simulink model "UAV_Research_Environment"  (R2025a)
settings: Solver=ode23t  StartTime=0.0  StopTime=130  MaxStep=2e-3  RelTol=1e-4  AbsTol=1e-3  EnableMultiTasking=on
InitFcn:
  | skipInitialization = false;
  | 
  | if evalin('base', ...
  |         'exist(''CONTROLLER_TUNING_ACTIVE'',''var'')')
  | 
  |     skipInitialization = evalin('base', ...
  |         'logical(CONTROLLER_TUNING_ACTIVE)');
  | end
  | 
  | if ~skipInitialization
  | 
  |     icraControllerPrepared = false;
  | 
  |     hasICRAVariables = evalin('base', ...
  |         ['exist(''AUTOPILOT'',''var'') && ' ...
  |          'exist(''ICRA_ACTIVE_CONTROLLER'',''var'') && ' ...
  |          'exist(''ICRA_ACTIVE_RUN_ID'',''var'')']);
  | 
  |     if hasICRAVariables
  | 
  |         icraControllerPrepared = evalin('base', ...
  |             ['isstruct(AUTOPILOT) && ' ...
  |              'isfield(AUTOPILOT,''info'') && ' ...
  |              'isfield(AUTOPILOT.info,''ICRAControllerID'') && ' ...
  |              'strcmp(string(AUTOPILOT.info.ICRAControllerID), ' ...
  |                     'string(ICRA_ACTIVE_CONTROLLER))']);
  | 
  |     end
  | 
  |     if icraControllerPrepared
  |         skipInitialization = true;
  |     end
  | end
  | 
  | if ~skipInitialization
  | 
  |     mdl = bdroot;
  | 
  |     mdl_file = get_param(mdl, 'FileName');
  | 
  |     project_root = fileparts(mdl_file);
  | 
  |     init_file = fullfile(project_root, 'initialize_project.m');
  | 
  |     if exist(init_file, 'file')
  | 
  |         run(init_file);
  | 
  |     else
  | 
  |         error('initialize_project.m was not found in the model folder.');
  | 
  |     end
  | end
values from neighbouring files (symbols this model uses):
  A_UAV = struct()    [UAV_analytical.m]
  AUTOPILOT = struct()    [UAV_autopilot.m]
  B_UAV = struct()    [UAV_block.m]
  D = A_UAV.source.propeller_diameter_m    [UAV_analytical.m]    (also in plot_controller_results.m = permute(                  D,                  order); plot_estimator_results.m = permute(              D,              order); plot_mission_results.m = permute(                  D,                  order); plot_touchdown_diagnostics.m = permute(                  D,                  order))
  OPERATOR_MODE = OPERATOR_MODE_MANUAL    [initialize_project.m]    (also in uav_remote_gui.m = uint8(0))
  P_ENV = struct()    [Environment.m]
  P_UAV = struct()    [UAV_simscape.m]
  s = sin(angle)    [uav_remote_gui.m]
  SENSOR = struct()    [UAV_sensors.m]
  TRAJECTORY_CONFIG = struct()    [UAV_trajectories.m]
  TRAJECTORY_ID = uint8(          trajectoryIDNumeric)    [UAV_trajectories.m]
  X = reshape(                  D,                  nt,                  [])    [plot_controller_results.m]    (also in plot_estimator_results.m = reshape(              D,              nt,              []); plot_mission_results.m; plot_touchdown_diagnostics.m; plot_trajectory_3d.m)
  Y = absolutePlanNED(1,:)    [plot_trajectory_3d.m]    (also in uav_remote_gui.m = positionNED(:,1))
  Z = landedCGDown -          absolutePlanNED(3,:)    [plot_trajectory_3d.m]    (also in uav_remote_gui.m = landedCGDown-positionNED(:,3))
undefined symbols (not defined in the file or in its folder): Acceleration_ref, F, fractalcoef, Light, MIL, Position_ref, Velocity_ref, Yaw_ref, YawRate_ref
libraries: sm_lib x49, nesl_utility x29, fl_lib x17, slpidlib x16, simulink x14, ee_lib x5, sdl_lib x4, aerolibwind2 x3, aerolibatmos2 x2, sensorbarometerlib x1, sensorgpslib x1, mspsensorlib x1
(part 1 of 9)
settings Model: ModifiedByFormat=Anonymous  Creator=Anonymous  LastModifiedBy=Anonymous
settings SolverCC: AutoScaleAbsTol=off  ZeroCrossAlgorithm=Adaptive  MaxZcPerStep=1.0
settings DataIOCC: LimitDataPoints=on  MaxDataPoints=10000  DSMLogging=off
settings OptimizationCC: ReuseModelBlockBuffer=off  LifeSpan=inf
settings DebuggingCC: AlgebraicLoopMsg=none  IgnoredZcDiagnostic=none  UnconnectedInputMsg=warning  UnconnectedOutputMsg=warning  UnconnectedLineMsg=warning  AllowSymbolicDim=off  SubsystemReferenceDiagnosticForUnitTest=warning  SFUnexpectedBacktrackingDiag=warning  SFNoUnconditionalDefaultTransitionDiag=warning  SFExecutionAtInitializationDiag=none  ArithmeticOperatorsInVariantConditions=warning
settings ModelReferenceCC: EnableRefExpFcnMdlSchedulingChecks=on
settings SFSimCC: SimUseLocalCustomCode=off  CustomCodeUndefinedFunction=UseInterfaceOnly
settings RTWCC: RTWUseLocalCustomCode=off  GPUComputeCapability=3.5  DLArmComputeVersion=19.05
settings CodeAppCC: StateflowObjectComments=on
settings GRTTargetCC: TargetLangStandard=C89/C90 (ANSI)
settings ConfigComp: CovMetricSettings=dw  CovSaveCumulativeToWorkspaceVar=on  CovSaveSingleToWorkspaceVar=on  CovExternalEMLEnable=off  CovSFcnEnable=off
settings SimscapeCC: SimscapeLogDataHistory=10000.0
settings ExplorerConfigSet: InternalSimMechanicsExplorerSettings=|
  | <ExplorerConfiguration>
  | 
  |   <canonicalview>default</canonicalview>
  | 
  |   <TilePanel>
  |     <TileInfo>
  |       <Tiles Columns="1" Count="1" Height="815" Rows="1" Width="1140">
  |         <Row Weight="1"/>
  |         <Column Weight="1"/>
  |         <Tile Height="1" Width="1" X="0" Y="0"/>
  |       </Tiles>
  |     </TileInfo>
  |     <SceneInfo>
  |       <SceneViewer>
  |         <IsThisViewStd>
  |           <IsStandardView>off</IsStandardView>
  |           <StandardViewName>Front</StandardViewName>
  |         </IsThisViewStd>
  |         <BGColor>
  |           <R>1</R>
  |           <G>1</G>
  |           <B>1</B>
  |           <A>1</A>
  |         </BGColor>
  |         <Camera>
  |           <DoPerspective>off</DoPerspective>
  |           <Position>
  |             <X>0.72021697851709687</X>
  |             <Y>23.914268823911655</Y>
  |             <Z>0.9247861603673575</Z>
  |           </Position>
  |           <Center>
  |             <X>0.72021697851709687</X>
  |             <Y>0.79760772389431911</Y>
  |             <Z>0.9247861603673575</Z>
  |           </Center>
  |           <Up>
  |             <X>0</X>
  |             <Y>0</Y>
  |             <Z>1</Z>
  |           </Up>
  |           <XLim>3.1326972550118835</XLim>
  |           <YLim>3.1326972550118835</YLim>
  |           <ViewLimDist>0.01</ViewLimDist>
  |         </Camera>
  |       </SceneViewer>
  |     </SceneInfo>
  |   </TilePanel>
  | 
  |   <MechEditorPanel>
  |     <GfxPanelCameraMap/>
  |     <Cameras/>
  |     <VideoCreator>
  |       <IncludeTiles>All</IncludeTiles>
  |       <IncludeTime>on</IncludeTime>
  |       <IncludeWorldFrame>off</IncludeWorldFrame>
  |       <PlaybackSpeedRatio>1</PlaybackSpeedRatio>
  |       <FrameRate>30</FrameRate>
  |       <FrameSize>auto</FrameSize>
  |       <VideoFormat>UncompressedAVI</VideoFormat>
  |     </VideoCreator>
  |   </MechEditorPanel>
  | 
  |   <PlaybackSettings>
  |     <PlaybackSpeedFactor>1</PlaybackSpeedFactor>
  |   </PlaybackSettings>
  | 
  | </ExplorerConfiguration>

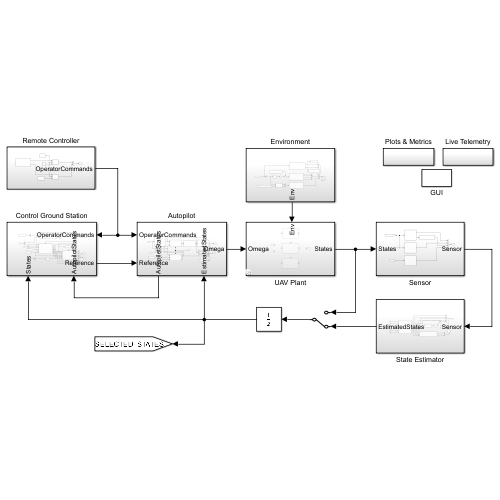
[thumbnail: Simulink's stored preview of the top-level diagram]
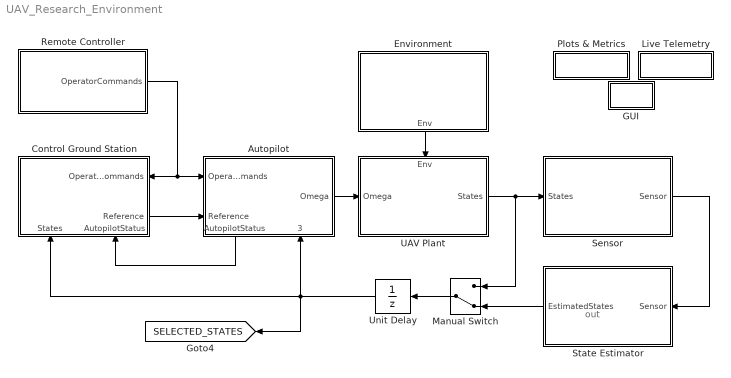
== system UAV_Research_Environment ==
  note: out
  Autopilot : Subsystem
      settings: PortSchema="{\"entries\":[{\"content\":{\"sides\":[{\"content\":{\"connectorIds\":[\"In1\",\"In2\"]},\"type\":\"ConnectorPlacement.EquallySpacedRectSide\",\"uuid\":\"e70f1091-d358-4451-85c8-8eba7ccb6162\"},{\"content\":{\"connectorIds\":[\"Out1\"],\"side\":\"RIGHT\"},\"type\":\"ConnectorPlacement.EquallySpacedRectSide\",\"uuid\":\"2dd7087d-b972-437c-8483-21f370874524\"},{\"content\":{\"side\":\"TOP\"},\"type\":\"ConnectorPlacement.EquallySpacedRectSide\",\"uuid\":\"61fa1c6d-d900-4918-8b03-2266ce99a694\"},{\"content\":{\"connectorIds\":[\"Out2\",\"In3\"],\"side\":\"BOTTOM\"},\"type\":\"ConnectorPlacement.EquallySpacedRectSide\",\"uuid\":\"0a489e47-d763-416d-8560-669941892c49\"}]},\"type\":\"ConnectorPlacement.EquallySpacedConnector\",\"uuid\":\"bc420e13-87ad-4ba2-aca7-0668641bff4a\"}],\"packageUris\":[\"http://schema.mathworks.com/mf0/Connector/R2020b\"],\"version\":\"1.0\"}"
  Control Ground Station : Subsystem
      settings: PortSchema="{\"entries\":[{\"content\":{\"sides\":[{\"content\":{},\"type\":\"ConnectorPlacement.EquallySpacedRectSide\",\"uuid\":\"136384be-95d6-4553-ba03-2aeaf9dd8964\"},{\"content\":{\"connectorIds\":[\"In3\",\"Out1\"],\"side\":\"RIGHT\"},\"type\":\"ConnectorPlacement.EquallySpacedRectSide\",\"uuid\":\"258859f6-93b5-427a-ab6d-3a33e6d3f50d\"},{\"content\":{\"side\":\"TOP\"},\"type\":\"ConnectorPlacement.EquallySpacedRectSide\",\"uuid\":\"470d9523-0035-468d-b4f0-7ce4b4aa87dd\"},{\"content\":{\"connectorIds\":[\"In1\",\"In2\"],\"side\":\"BOTTOM\"},\"type\":\"ConnectorPlacement.EquallySpacedRectSide\",\"uuid\":\"eb9250ba-ba34-48b7-bfa4-7567789009ef\"}]},\"type\":\"ConnectorPlacement.EquallySpacedConnector\",\"uuid\":\"8818c9e9-852d-490b-83ee-80294e50417b\"}],\"packageUris\":[\"http://schema.mathworks.com/mf0/Connector/R2020b\"],\"version\":\"1.0\"}"
  Environment : Subsystem
      settings: PortSchema="{\"entries\":[{\"content\":{\"sides\":[{\"content\":{},\"type\":\"ConnectorPlacement.EquallySpacedRectSide\",\"uuid\":\"20d534b3-ad30-4c14-921c-ffe2bc2505b4\"},{\"content\":{\"side\":\"RIGHT\"},\"type\":\"ConnectorPlacement.EquallySpacedRectSide\",\"uuid\":\"42e7d556-7bdf-4888-9f8c-71685b18f3c6\"},{\"content\":{\"side\":\"TOP\"},\"type\":\"ConnectorPlacement.EquallySpacedRectSide\",\"uuid\":\"98b28398-80a3-4874-ba79-5e078ee713b6\"},{\"content\":{\"connectorIds\":[\"Out1\"],\"side\":\"BOTTOM\"},\"type\":\"ConnectorPlacement.EquallySpacedRectSide\",\"uuid\":\"66822910-7c6b-4720-98d4-5d952560352f\"}]},\"type\":\"ConnectorPlacement.EquallySpacedConnector\",\"uuid\":\"f342a492-18c2-4fcb-af45-73348ac80d72\"}],\"packageUris\":[\"http://schema.mathworks.com/mf0/Connector/R2020b\"],\"version\":\"1.0\"}"
  GUI : Subsystem
      settings: OpenFcn=|
      | mdl = bdroot(gcb);
      | mdlFolder = fileparts(get_param(mdl,'FileName'));
      | 
      | oldFolder = pwd;
      | cleanupObj = onCleanup(@() cd(oldFolder));
      | 
      | cd(mdlFolder);
      | uav_remote_gui(mdl);
  Live Telemetry : Subsystem
  Manual Switch : ManualSwitch  CurrentSetting=0
  Plots & Metrics : Subsystem
  Remote Controller : Subsystem
  Sensor : Subsystem
  State Estimator : Subsystem
      settings: PortSchema="{\"entries\":[{\"content\":{\"sides\":[{\"content\":{\"connectorIds\":[\"Out1\"]},\"type\":\"ConnectorPlacement.EquallySpacedRectSide\",\"uuid\":\"59a621b8-c7fd-4210-ae06-7e4287b99fe9\"},{\"content\":{\"connectorIds\":[\"In1\"],\"side\":\"RIGHT\"},\"type\":\"ConnectorPlacement.EquallySpacedRectSide\",\"uuid\":\"3b6e64c1-8f25-466d-be87-51a5dfb932f3\"},{\"content\":{\"side\":\"TOP\"},\"type\":\"ConnectorPlacement.EquallySpacedRectSide\",\"uuid\":\"7168969e-7eff-41f7-8f21-8d68bf623552\"}]},\"type\":\"ConnectorPlacement.EquallySpacedConnector\",\"uuid\":\"8e25eed9-214a-4c11-975e-8e28997d468c\"}],\"packageUris\":[\"http://schema.mathworks.com/mf0/Connector/R2020b\"],\"version\":\"1.0\"}"
  UAV Plant : Subsystem  Variant=on  AllowFlexibleInterface=off
      settings: PortSchema="{\"entries\":[{\"content\":{\"sides\":[{\"content\":{\"connectorIds\":[\"In1\"]},\"type\":\"ConnectorPlacement.EquallySpacedRectSide\",\"uuid\":\"3610bc50-1c95-4e4a-95b0-008058f44424\"},{\"content\":{\"connectorIds\":[\"Out1\"],\"side\":\"RIGHT\"},\"type\":\"ConnectorPlacement.EquallySpacedRectSide\",\"uuid\":\"eac11400-6209-4713-b6ed-f17afc459a7e\"},{\"content\":{\"connectorIds\":[\"In2\"],\"side\":\"TOP\"},\"type\":\"ConnectorPlacement.EquallySpacedRectSide\",\"uuid\":\"1cd5a0d1-33ba-4090-85ff-88440ab8bf38\"}]},\"type\":\"ConnectorPlacement.EquallySpacedConnector\",\"uuid\":\"d77e6d8a-bf97-49e4-8cac-05db6bcacb57\"}],\"packageUris\":[\"http://schema.mathworks.com/mf0/Connector/R2020b\"],\"version\":\"1.0\"}"
  Unit Delay : UnitDelay  SampleTime=-1  HasFrameUpgradeWarning=on
  tag scope: SELECTED_STATES=global
  wires:
  UAV Plant/1(States) -> Sensor/1(States), Manual Switch/1
  Sensor/1(Sensor) -> State Estimator/1(Sensor)
  Control Ground Station/1(Reference) -> Autopilot/2(Reference)
  Remote Controller/1(OperatorCommands) -> Control Ground Station/3(OperatorCommands), Autopilot/1(OperatorCommands)
  Autopilot/2(AutopilotStatus) -> Control Ground Station/2(AutopilotStatus)
  Manual Switch/1 -> Unit Delay/1
  Unit Delay/1 -> Control Ground Station/1(States), Autopilot/3(EstimatedStates), [SELECTED_STATES]
  State Estimator/1(EstimatedStates) -> Manual Switch/2
  Autopilot/1(Omega) -> UAV Plant/1(Omega)
  Environment/1(Env) -> UAV Plant/2(Env)

== system UAV_Research_Environment/Autopilot ==
  OperatorCommands : Inport
  Reference : Inport  Port=2
  EstimatedStates : Inport  Port=3
  Bus Creator : BusCreator  Inputs=5
  Bus Selector : BusSelector  OutputSignals=mode,armed,reset,missionComplete
  Control Allocation : Subsystem
  Flight Control : Subsystem
      settings: PortSchema="{\"entries\":[{\"content\":{\"sides\":[{\"content\":{\"connectorIds\":[\"In1\",\"In2\"]},\"type\":\"ConnectorPlacement.EquallySpacedRectSide\",\"uuid\":\"f0a7248d-f68a-4ef2-8432-35dfc7f6e14f\"},{\"content\":{\"connectorIds\":[\"Out1\"],\"side\":\"RIGHT\"},\"type\":\"ConnectorPlacement.EquallySpacedRectSide\",\"uuid\":\"efba777c-49ac-415f-93a0-e17947ba5c8f\"},{\"content\":{\"side\":\"TOP\"},\"type\":\"ConnectorPlacement.EquallySpacedRectSide\",\"uuid\":\"6197b28d-1ee2-4df8-818f-0bd555e896ae\"},{\"content\":{\"connectorIds\":[\"In3\"],\"side\":\"BOTTOM\"},\"type\":\"ConnectorPlacement.EquallySpacedRectSide\",\"uuid\":\"82eb3d58-e8e8-4a8e-8208-c30c9bf3b54b\"}]},\"type\":\"ConnectorPlacement.EquallySpacedConnector\",\"uuid\":\"801f385a-c387-4f85-8315-b8cc9b2ee46f\"}],\"packageUris\":[\"http://schema.mathworks.com/mf0/Connector/R2020b\"],\"version\":\"1.0\"}"
  Flight Management : Subsystem
      settings: PortSchema="{\"entries\":[{\"content\":{\"sides\":[{\"content\":{\"connectorIds\":[\"In1\"]},\"type\":\"ConnectorPlacement.EquallySpacedRectSide\",\"uuid\":\"cd28ed6d-ec01-4006-9fc1-ea9cf3b5ab9c\"},{\"content\":{\"connectorIds\":[\"Out1\"],\"side\":\"RIGHT\"},\"type\":\"ConnectorPlacement.EquallySpacedRectSide\",\"uuid\":\"9cadd399-a218-43e8-9df1-ffad97f9a650\"},{\"content\":{\"side\":\"TOP\"},\"type\":\"ConnectorPlacement.EquallySpacedRectSide\",\"uuid\":\"feac389c-df1b-4914-811b-4035f0dee4d7\"},{\"content\":{\"connectorIds\":[\"In2\",\"In3\",\"In4\",\"In5\"],\"side\":\"BOTTOM\"},\"type\":\"ConnectorPlacement.EquallySpacedRectSide\",\"uuid\":\"4a7ea741-3b46-4c9a-969c-f6d865221263\"}]},\"type\":\"ConnectorPlacement.EquallySpacedConnector\",\"uuid\":\"336e0f35-9a21-4036-b176-5dadcac79355\"}],\"packageUris\":[\"http://schema.mathworks.com/mf0/Connector/R2020b\"],\"version\":\"1.0\"}"
  Landed Detector : Subsystem
      settings: PortSchema="{\"entries\":[{\"content\":{\"sides\":[{\"content\":{\"connectorIds\":[\"In1\",\"In2\",\"In3\"]},\"type\":\"ConnectorPlacement.EquallySpacedRectSide\",\"uuid\":\"9d9528e8-7e55-467e-913b-dcdc8299219a\"},{\"content\":{\"connectorIds\":[\"Out1\",\"Out2\"],\"side\":\"RIGHT\"},\"type\":\"ConnectorPlacement.EquallySpacedRectSide\",\"uuid\":\"a2ddb638-2a20-4bf0-9798-8e8fe050fb6e\"},{\"content\":{\"connectorIds\":[\"In4\"],\"side\":\"TOP\"},\"type\":\"ConnectorPlacement.EquallySpacedRectSide\",\"uuid\":\"4b4cf5b5-d356-42f7-9123-fe3c672c98b7\"}]},\"type\":\"ConnectorPlacement.EquallySpacedConnector\",\"uuid\":\"5fd14821-3580-4c60-a331-c7350594f720\"}],\"packageUris\":[\"http://schema.mathworks.com/mf0/Connector/R2020b\"],\"version\":\"1.0\"}"
  Motor Command : Subsystem
      settings: PortSchema="{\"entries\":[{\"content\":{\"sides\":[{\"content\":{\"connectorIds\":[\"In1\"]},\"type\":\"ConnectorPlacement.EquallySpacedRectSide\",\"uuid\":\"f0a7248d-f68a-4ef2-8432-35dfc7f6e14f\"},{\"content\":{\"connectorIds\":[\"Out1\"],\"side\":\"RIGHT\"},\"type\":\"ConnectorPlacement.EquallySpacedRectSide\",\"uuid\":\"efba777c-49ac-415f-93a0-e17947ba5c8f\"},{\"content\":{\"connectorIds\":[\"In2\"],\"side\":\"TOP\"},\"type\":\"ConnectorPlacement.EquallySpacedRectSide\",\"uuid\":\"6197b28d-1ee2-4df8-818f-0bd555e896ae\"}]},\"type\":\"ConnectorPlacement.EquallySpacedConnector\",\"uuid\":\"801f385a-c387-4f85-8315-b8cc9b2ee46f\"}],\"packageUris\":[\"http://schema.mathworks.com/mf0/Connector/R2020b\"],\"version\":\"1.0\"}"
  Omega : Outport
  AutopilotStatus : Outport  Port=2
  tag scope: AUTOPILOT_ST=global, OMEGA=global
  wires:
  Flight Control/1(FlightControl) -> Control Allocation/1(FlightControl)
  Control Allocation/1(MotorCmd) -> Motor Command/1(MotorCmd)
  Motor Command/1(Omega) -> Omega/1, [OMEGA]
  Flight Management/1(FlightManagement) -> Bus Selector/1, Motor Command/2(FlightManagement), Flight Control/1(FlightManagement)
  Reference/1 -> Landed Detector/1(Reference), Flight Control/2(Reference), Flight Management/1(Reference)
  EstimatedStates/1 -> Flight Control/3(EstimatedStates), Landed Detector/4(EstimatedStates)
  OperatorCommands/1 -> Landed Detector/3(OperatorCommands), Flight Management/3(OperatorCommands)
  Landed Detector/1(Landed) -> Flight Management/2(Landed), Bus Creator/5  "Landed"
  Bus Selector/1 -> Bus Creator/1  "<mode>"
  Bus Selector/2 -> Bus Creator/2  "<armed>"
  Bus Selector/3 -> Bus Creator/3  "<reset>"
  Bus Selector/4 -> Bus Creator/4  "<missionComplete>"
  Bus Creator/1 -> [AUTOPILOT_ST], AutopilotStatus/1
  [EST_STATUS] -> Flight Management/4(EstimatorStatus), Landed Detector/2(EstimatorStatus)
  Landed Detector/2(TouchdownCandidate) -> Flight Management/5(TouchdownCandidate)

== system UAV_Research_Environment/Control Ground Station ==
  States : Inport
  AutopilotStatus : Inport  Port=2
  OperatorCommands : Inport  Port=3
  Bus Creator : BusCreator  Inputs=8
  Bus Selector : BusSelector  OutputSignals=ArmCommand,RunTrajectoryRequestID
  Bus Selector1 : BusSelector  OutputSignals=Position,Velocity
  Bus Selector2 : BusSelector  OutputSignals=Landed
  Bus Selector3 : BusSelector  OutputSignals=Position
  "Digital Clock " : DigitalClock  SampleTime=AUTOPILOT.rate.controlSampleTime_s
  Home Manager : MATLAB Function  TreatAsAtomicUnit=on
  Mission Manager : Subsystem
      settings: PortSchema="{\"entries\":[{\"content\":{\"sides\":[{\"content\":{\"connectorIds\":[\"In1\",\"In2\",\"In3\",\"In4\",\"In5\",\"In6\"]},\"type\":\"ConnectorPlacement.EquallySpacedRectSide\",\"uuid\":\"bc5e4697-56b9-4dea-9e35-80b1d53c2be1\"},{\"content\":{\"connectorIds\":[\"Out1\",\"Out2\",\"Out3\",\"Out4\",\"Out5\",\"Out6\"],\"side\":\"RIGHT\"},\"type\":\"ConnectorPlacement.EquallySpacedRectSide\",\"uuid\":\"fb3706cb-7914-4411-8945-e3646c2cb779\"},{\"content\":{\"connectorIds\":[\"In7\"],\"side\":\"TOP\"},\"type\":\"ConnectorPlacement.EquallySpacedRectSide\",\"uuid\":\"dbed3f0a-ac38-4c4a-aeac-a7a9b73a6d14\"}]},\"type\":\"ConnectorPlacement.EquallySpacedConnector\",\"uuid\":\"9e38a936-7e60-4815-89b3-1f8eea1eae0e\"}],\"packageUris\":[\"http://schema.mathworks.com/mf0/Connector/R2020b\"],\"version\":\"1.0\"}"
  Mission Plan : Subsystem
  Terminator : Terminator
  Unit Delay : UnitDelay  InitialCondition=false  SampleTime=0.005  HasFrameUpgradeWarning=on
  Waypoint Navigator : Subsystem
      settings: PortSchema="{\"entries\":[{\"content\":{\"sides\":[{\"content\":{\"connectorIds\":[\"In1\",\"In2\",\"In3\",\"In4\",\"In5\",\"In6\",\"In7\"]},\"type\":\"ConnectorPlacement.EquallySpacedRectSide\",\"uuid\":\"a5c6b6ee-d5d5-4725-a074-dc49922cc7be\"},{\"content\":{\"connectorIds\":[\"Out1\",\"Out2\",\"Out3\",\"Out4\",\"Out5\"],\"side\":\"RIGHT\"},\"type\":\"ConnectorPlacement.EquallySpacedRectSide\",\"uuid\":\"658ed11c-ff5e-46da-8e6b-259d14db485f\"},{\"content\":{\"connectorIds\":[\"In8\"],\"side\":\"TOP\"},\"type\":\"ConnectorPlacement.EquallySpacedRectSide\",\"uuid\":\"7f46b370-90bd-452a-8751-2617752800df\"}]},\"type\":\"ConnectorPlacement.EquallySpacedConnector\",\"uuid\":\"a0f43945-89fe-4e34-a980-6cf45089d260\"}],\"packageUris\":[\"http://schema.mathworks.com/mf0/Connector/R2020b\"],\"version\":\"1.0\"}"
  Reference : Outport
  tag scope: CGS=global, MISSION_PLAN=global, NUM_WAYPOINTS=global
  wires:
  OperatorCommands/1 -> Bus Selector/1
  Bus Selector/2 -> Mission Manager/1(RunTrajectoryRequestID)  "<RunTrajectoryRequestID>"
  States/1 -> Bus Selector1/1
  Bus Selector1/2 -> Mission Manager/3(Velocity)  "<Velocity>"
  "Digital Clock "/1 -> Waypoint Navigator/1(t), Mission Manager/6(t)
  Bus Selector1/1 -> Mission Manager/2(Position)  "<Position>"
  Mission Manager/1(TargetPosition) -> Waypoint Navigator/3(TargetPosition)
  Mission Manager/2(TargetYaw) -> Waypoint Navigator/4(TargetYaw)
  Mission Manager/3(TargetID) -> Waypoint Navigator/5(TargetID)
  Bus Creator/1 -> [CGS], Reference/1
  Waypoint Navigator/1(Position_ref) -> Bus Creator/1
  Waypoint Navigator/2(Velocity_ref) -> Bus Creator/2
  Waypoint Navigator/3(Acceleration_ref) -> Bus Creator/3
  Waypoint Navigator/4(Yaw_ref) -> Bus Creator/4
  Waypoint Navigator/5(YawRate_ref) -> Bus Creator/5
  Mission Manager/4(Phase) -> Bus Creator/6, Waypoint Navigator/6(Phase)
  Mission Manager/5(Active) -> Bus Creator/7
  Mission Manager/6(Complete) -> Bus Creator/8
  AutopilotStatus/1 -> Bus Selector2/1
  Bus Selector2/1 -> Unit Delay/1  "<Landed>"
  Unit Delay/1 -> Waypoint Navigator/7(Landed)
  Bus Selector/1 -> Home Manager/2(ArmCommand)  "<ArmCommand>"
  Home Manager/1(HomePosition) -> Mission Plan/1(HomePosition)
  [EST_STATUS] -> Mission Manager/4(EstimatorStatus)
  Mission Plan/1(MissionPlan) -> Waypoint Navigator/2(MissionPlan), [MISSION_PLAN], Mission Manager/7(MissionPlan)
  [TRUE_STATES] -> Bus Selector3/1
  Bus Selector3/1 -> Home Manager/1(HomePositionSource)  "<Position>"
  Mission Plan/2(NumWaypoints) -> [NUM_WAYPOINTS], Waypoint Navigator/8(NumWaypoints), Mission Manager/5(NumWaypoints)
  Home Manager/2(HomeValid) -> Terminator/1

== system UAV_Research_Environment/Environment ==
  Atmosphere : aerolibatmos2/ISA Atmosphere Model  useExtended=off  action=None  custom=off  viscosityOut=off  g=9.80665  gamma=1.4  R=287.0531  L=0.0065  h_trop=11000  h_strat=20000  rho0=1.225  P0=101325  T0=288.15  h0=0  S=110.4  Tref=273.15  muref=1.716e-5
  Bus Creator : BusCreator  Inputs=3
  Bus Creator1 : BusCreator  Inputs=2
  Bus Creator2 : BusCreator  Inputs=4
  Bus Selector2 : BusSelector  OutputSignals=Position
  Constant : Constant  Value=P_ENV.location.altitude_ref_m
  Constant1 : Constant  Value=P_ENV.location.flat_earth_href_m
  Flat Earth to LLA : FlatEarth2LLA  LL0=[P_ENV.location.latitude_ref_deg P_ENV.location.longitude_ref_deg]  psi=P_ENV.location.heading_ref_deg
  Gain : Gain  Gain=-1
  Gravity : GravityWGS84
  Selector : Selector  InputPortWidth=3  IndexOptions=Index vector (dialog)  Indices=3  OutputSizes=1
  Sum : Sum  Inputs=++|
  To Workspace : ToWorkspace  VariableName=windVelocityLog  SaveFormat=Timeseries  SampleTime=-1
  To Workspace1 : ToWorkspace  VariableName=windAngularVelocityLog  SaveFormat=Timeseries  SampleTime=-1
  Vector Concatenate1 : Concatenate
  Wind Disturbances : Subsystem  Variant=on
  Env : Outport
  tag scope: ENV=global
  wires:
  Gain/1 -> Sum/2
  Wind Disturbances/1(v_wind) -> Bus Creator1/1, To Workspace/1  "v"
  Atmosphere/1 -> Bus Creator2/1  "Temperature"
  Atmosphere/2 -> Bus Creator2/2  "SoundSpeed"
  Atmosphere/4 -> Bus Creator2/4  "AirDensity"
  Atmosphere/3 -> Bus Creator2/3  "AirPressure"
  Gravity/1 -> Bus Creator/3  "Gravity"
  [TRUE_STATES] -> Wind Disturbances/1(States), Bus Selector2/1
  Constant1/1 -> Flat Earth to LLA/2
  Flat Earth to LLA/1 -> Vector Concatenate1/1
  Flat Earth to LLA/2 -> Vector Concatenate1/2
  Vector Concatenate1/1 -> Gravity/1
  Bus Selector2/1 -> Selector/1, Flat Earth to LLA/1  "<Position>"
  Wind Disturbances/2(w_wind) -> Bus Creator1/2, To Workspace1/1  "w"
  Selector/1 -> Gain/1  "z"
  Bus Creator/1 -> Env/1, [ENV]
  Bus Creator2/1 -> Bus Creator/2  "Atmosphere"
  Bus Creator1/1 -> Bus Creator/1  "Wind"
  Sum/1 -> Atmosphere/1
  Constant/1 -> Sum/1

== system UAV_Research_Environment/GUI ==

== system UAV_Research_Environment/Live Telemetry ==
  Bus Selector : BusSelector  OutputSignals=Phase,Active,Complete,Position_ref
  Bus Selector1 : BusSelector  OutputSignals=Position,Attitude.Euler
  Bus Selector2 : BusSelector  OutputSignals=mode,armed,missionComplete,Landed
  Bus Selector3 : BusSelector  OutputSignals=Position,Attitude.Euler
  Bus Selector4 : BusSelector  OutputSignals=Position
  "Digital Clock " : DigitalClock  SampleTime=AUTOPILOT.rate.controlSampleTime_s
  Telemetry_Pack : MATLAB Function  TreatAsAtomicUnit=on
  To Workspace : ToWorkspace  VariableName=liveTelemetryLog  SaveFormat=Timeseries  SampleTime=-1
  wires:
  [CGS] -> Bus Selector/1
  [SELECTED_STATES] -> Bus Selector1/1
  [AUTOPILOT_ST] -> Bus Selector2/1
  "Digital Clock "/1 -> Telemetry_Pack/1(t)
  Bus Selector/1 -> Telemetry_Pack/2(Phase)  "<Phase>"
  Bus Selector/2 -> Telemetry_Pack/3(Active)  "<Active>"
  Bus Selector/3 -> Telemetry_Pack/4(Complete)  "<Complete>"
  Bus Selector/4 -> Telemetry_Pack/5(Position_ref)  "<Position_ref>"
  Bus Selector1/1 -> Telemetry_Pack/10(Position)  "<Position>"
  Bus Selector2/1 -> Telemetry_Pack/6(mode)  "<mode>"
  Bus Selector2/2 -> Telemetry_Pack/7(armed)  "<armed>"
  Bus Selector2/3 -> Telemetry_Pack/8(missionComplete)  "<missionComplete>"
  Bus Selector2/4 -> Telemetry_Pack/9(Landed)  "<Landed>"
  Telemetry_Pack/1(Telemetry) -> To Workspace/1
  [MISSION_PLAN] -> Telemetry_Pack/13(MissionPlan)
  [OMEGA] -> Telemetry_Pack/12(MotorSpeeds)
  Bus Selector1/2 -> Telemetry_Pack/11(Euler)  "<Euler>"
  [TRUE_STATES] -> Bus Selector3/1
  [EST_STATES] -> Bus Selector4/1
  Bus Selector4/1 -> Telemetry_Pack/16(EstPosition)  "<Position>"
  Bus Selector3/2 -> Telemetry_Pack/15(TrueEuler)  "<Euler>"
  Bus Selector3/1 -> Telemetry_Pack/14(TruePosition)  "<Position>"
  [NUM_WAYPOINTS] -> Telemetry_Pack/17(NumWaypoints)

== system UAV_Research_Environment/Plots & Metrics ==
  Data Logging : Subsystem
  Estimator Comparison : Subsystem
  wires:
  [TRUE_STATES] -> Data Logging/3(TrueStates), Estimator Comparison/1(True)
  [EST_STATES] -> Data Logging/2(EstStates), Estimator Comparison/2(Est)
  Estimator Comparison/1(EstimatorComparison) -> Data Logging/1(EstimatorComparison)
  [CGS] -> Data Logging/7(CGS)
  [OMEGA] -> Data Logging/4(Omega)
  [CONTROL_AXES] -> Data Logging/5(ControlAxes)
  [CMD_ATTITUDE] -> Data Logging/6(CmdAttitude)
  [CMD_ANGULAR_RATE] -> Data Logging/8(CmdAngularRate)
  [SELECTED_STATES] -> Data Logging/9(SelectedStates)
  [MISSION_PLAN] -> Data Logging/10("MissionPlan ")

== system UAV_Research_Environment/Remote Controller ==
  Arm Command : Constant  Value=false  OutDataTypeStr=boolean  SampleTime=AUTOPILOT.rate.controlSampleTime_s
  Arm Selector : Switch  Criteria=u2 ~= 0  Threshold=0.5  SaturateOnIntegerOverflow=off  InputSameDT=off
  Automatic Operator : Subsystem
  Bus Creator : BusCreator  Inputs=2
  Operator Mode : Constant  Value=OPERATOR_MODE  OutDataTypeStr=uint8
  Run Selector : Switch  Criteria=u2 ~= 0  Threshold=0.5  SaturateOnIntegerOverflow=off  InputSameDT=off
  Run Trajectory Request ID : Constant  Value=uint32(0)
  OperatorCommands : Outport
  wires:
  Arm Command/1 -> Arm Selector/3
  Automatic Operator/1(ArmCommand) -> Arm Selector/1  "Automatic Operator"
  Operator Mode/1 -> Run Selector/2, Arm Selector/2
  Bus Creator/1 -> OperatorCommands/1
  Arm Selector/1 -> Bus Creator/1  "ArmCommand"
  Run Selector/1 -> Bus Creator/2  "RunTrajectoryRequestID"
  Automatic Operator/2(RunTrajectoryRequestID) -> Run Selector/1  "RunTrajectoryRequestID"
  Run Trajectory Request ID/1 -> Run Selector/3

== system UAV_Research_Environment/Sensor ==
  States : Inport
  Barometer : Subsystem
  Bus Creator : BusCreator  Inputs=4
  GPS : Subsystem
  IMU : Subsystem
  Magnetometer : Subsystem
  Sensor : Outport
  tag scope: TRUE_STATES=global
  wires:
  States/1 -> GPS/1(States), [TRUE_STATES], IMU/1(States)
  [ENV] -> Barometer/1(Env)
  IMU/2(MagneticField) -> Magnetometer/1(MagneticField)
  IMU/1(IMU) -> Bus Creator/1  "IMU"
  GPS/1(GPS) -> Bus Creator/2  "GPS"
  Magnetometer/1(Magnetometer) -> Bus Creator/3  "Magnetometer"
  Barometer/1(Barometer) -> Bus Creator/4  "Barometer"
  Bus Creator/1 -> Sensor/1

== system UAV_Research_Environment/State Estimator ==
  Sensor : Inport
  Bus Creator : BusCreator  Inputs=5
  Bus Creator1 : BusCreator  Inputs=2
  Bus Creator2 : BusCreator  Inputs=2
  Bus Selector : BusSelector  OutputSignals=IMU.Accel,IMU.Gyro,GPS.LLA,Magnetometer.MagneticField,GPS.Velocity,Barometer.Altitude
  INS_EKF : MATLAB Function  TreatAsAtomicUnit=on
  Navigation_Health : MATLAB Function  TreatAsAtomicUnit=on
  Quaternions to Rotation Angles : Quat2Angle
      settings: AttributesFormatString=Rotation Order: %<rotationOrder>
  Selector : Selector  InputPortWidth=3  IndexOptions=Index vector (dialog)  Indices=[3 2 1]  OutputSizes=1
  Terminator : Terminator
  Terminator1 : Terminator
  Terminator2 : Terminator
  Unit Delay : UnitDelay  SampleTime=-1  HasFrameUpgradeWarning=on
  EstimatedStates : Outport
  tag scope: EST_STATES=global, EST_STATUS=global
  wires:
  Sensor/1 -> Bus Selector/1
  Bus Selector/1 -> INS_EKF/1(Accel)  "<Accel>"
  Bus Selector/2 -> INS_EKF/2(Gyro)  "<Gyro>"
  Bus Selector/4 -> INS_EKF/4(MagneticField)  "<MagneticField>"
  Bus Selector/6 -> INS_EKF/6(BaroAltitude)  "<Altitude>"
  Bus Selector/5 -> INS_EKF/5(GPSVelocity)  "<Velocity>"
  Bus Selector/3 -> INS_EKF/3(LLA)  "<LLA>"
  Bus Creator/1 -> EstimatedStates/1, [EST_STATES]
  INS_EKF/1(Position) -> Bus Creator/1
  INS_EKF/2(Velocity) -> Bus Creator/2
  INS_EKF/5(Acceleration) -> Bus Creator/3  "Acceleration"
  INS_EKF/4(AngularRate) -> Bus Creator/4  "AngularRate"
  Bus Creator1/1 -> Bus Creator/5  "Attitude"
  INS_EKF/3(Q) -> Quaternions to Rotation Angles/1, Bus Creator1/1  "Q"
  Quaternions to Rotation Angles/1 -> Selector/1
  Selector/1 -> Bus Creator1/2  "Euler"
  INS_EKF/9(HealthFlags) -> Navigation_Health/1(HealthFlags)  "HealthFlags"
  INS_EKF/10(StateStd) -> Navigation_Health/2(StateStd)  "StateStd"
  INS_EKF/11(InnovationSigma) -> Navigation_Health/3(InnovationSigma)  "InnovationSigma"
  Navigation_Health/1(NavValid) -> Bus Creator2/1  "NavValid"
  Navigation_Health/2(NavHealthStatus) -> Bus Creator2/2  "NavHealthStatus"
  Bus Creator2/1 -> Unit Delay/1
  Unit Delay/1 -> [EST_STATUS]
  INS_EKF/8(MagBias) -> Terminator2/1  "MagBias"
  INS_EKF/7(AccelBias) -> Terminator1/1  "AccelBias"
  INS_EKF/6(GyroBias) -> Terminator/1  "GyroBias"

== system UAV_Research_Environment/UAV Plant ==
  Omega : Inport
  Env : Inport  Port=2
  UAV Analytical [ODEs] : Subsystem  VariantControl=UAV_MODEL == 1
      settings: PortSchema="{\"entries\":[{\"content\":{\"sides\":[{\"content\":{\"connectorIds\":[\"In1\"]},\"type\":\"ConnectorPlacement.EquallySpacedRectSide\",\"uuid\":\"3610bc50-1c95-4e4a-95b0-008058f44424\"},{\"content\":{\"connectorIds\":[\"Out1\"],\"side\":\"RIGHT\"},\"type\":\"ConnectorPlacement.EquallySpacedRectSide\",\"uuid\":\"eac11400-6209-4713-b6ed-f17afc459a7e\"},{\"content\":{\"connectorIds\":[\"In2\"],\"side\":\"TOP\"},\"type\":\"ConnectorPlacement.EquallySpacedRectSide\",\"uuid\":\"1cd5a0d1-33ba-4090-85ff-88440ab8bf38\"}]},\"type\":\"ConnectorPlacement.EquallySpacedConnector\",\"uuid\":\"d77e6d8a-bf97-49e4-8cac-05db6bcacb57\"}],\"packageUris\":[\"http://schema.mathworks.com/mf0/Connector/R2020b\"],\"version\":\"1.0\"}"
  UAV Block [Simulink Blocks] : Subsystem  VariantControl=UAV_MODEL == 2
      settings: PortSchema="{\"entries\":[{\"content\":{\"sides\":[{\"content\":{\"connectorIds\":[\"In1\"]},\"type\":\"ConnectorPlacement.EquallySpacedRectSide\",\"uuid\":\"3610bc50-1c95-4e4a-95b0-008058f44424\"},{\"content\":{\"connectorIds\":[\"Out1\"],\"side\":\"RIGHT\"},\"type\":\"ConnectorPlacement.EquallySpacedRectSide\",\"uuid\":\"eac11400-6209-4713-b6ed-f17afc459a7e\"},{\"content\":{\"connectorIds\":[\"In2\"],\"side\":\"TOP\"},\"type\":\"ConnectorPlacement.EquallySpacedRectSide\",\"uuid\":\"1cd5a0d1-33ba-4090-85ff-88440ab8bf38\"}]},\"type\":\"ConnectorPlacement.EquallySpacedConnector\",\"uuid\":\"d77e6d8a-bf97-49e4-8cac-05db6bcacb57\"}],\"packageUris\":[\"http://schema.mathworks.com/mf0/Connector/R2020b\"],\"version\":\"1.0\"}"
  UAV Physical [Simscape] : Subsystem  VariantControl=UAV_MODEL == 3
      settings: PortSchema="{\"entries\":[{\"content\":{\"sides\":[{\"content\":{\"connectorIds\":[\"In1\"]},\"type\":\"ConnectorPlacement.EquallySpacedRectSide\",\"uuid\":\"cd72d1cb-8411-4d8b-9c3b-d51e45cdf4f4\"},{\"content\":{\"connectorIds\":[\"Out1\"],\"side\":\"RIGHT\"},\"type\":\"ConnectorPlacement.EquallySpacedRectSide\",\"uuid\":\"72bd53fa-ed96-4c13-8810-eb702aa341f9\"},{\"content\":{\"connectorIds\":[\"In2\"],\"side\":\"TOP\"},\"type\":\"ConnectorPlacement.EquallySpacedRectSide\",\"uuid\":\"724d920b-5c04-4257-b98a-9f6b1b16497a\"}]},\"type\":\"ConnectorPlacement.EquallySpacedConnector\",\"uuid\":\"a7b6d37f-3c60-453a-967a-9b7599e9c57f\"}],\"packageUris\":[\"http://schema.mathworks.com/mf0/Connector/R2020b\"],\"version\":\"1.0\"}"
  States : Outport

== system UAV_Research_Environment/Autopilot/Control Allocation ==
  FlightControl : Inport
  Bus Selector : BusSelector  OutputSignals=rollAxis,pitchAxis,yawAxis,thrustAxis
  Collective Thrust Distribution : Gain  Gain=AUTOPILOT.allocation.collectiveVector  Multiplication=Matrix(K*u)
  Effective Matrix Quadrotor : Constant  Value=AUTOPILOT.allocation.effectiveMatrix
  Hover Trim Omega : Constant  Value=AUTOPILOT.allocation.omegaTrim_rad_s
  Matrix Multiply : Product  Multiplication=Matrix(*)
  Mux : Mux  Inputs=3
  Sum : Sum  Inputs=+++
  MotorCmd : Outport
  tag scope: CONTROL_AXES=global
  wires:
  FlightControl/1 -> [CONTROL_AXES], Bus Selector/1
  Bus Selector/1 -> Mux/1  "<rollAxis>"
  Bus Selector/2 -> Mux/2  "<pitchAxis>"
  Bus Selector/3 -> Mux/3  "<yawAxis>"
  Bus Selector/4 -> Collective Thrust Distribution/1  "<thrustAxis>"
  Matrix Multiply/1 -> Sum/2  "MotorDifferential"
  Effective Matrix Quadrotor/1 -> Matrix Multiply/1
  Sum/1 -> MotorCmd/1
  Collective Thrust Distribution/1 -> Sum/3  "CollectiveCmd"
  Hover Trim Omega/1 -> Sum/1
  Mux/1 -> Matrix Multiply/2

== system UAV_Research_Environment/Autopilot/Flight Control ==
  FlightManagement : Inport
  Reference : Inport  Port=2
  EstimatedStates : Inport  Port=3
  Bus Creator : BusCreator  Inputs=4
  Controller Supervisor : Subsystem
  Error Computation : Subsystem
      settings: PortSchema="{\"entries\":[{\"content\":{\"sides\":[{\"content\":{\"connectorIds\":[\"In1\"]},\"type\":\"ConnectorPlacement.EquallySpacedRectSide\",\"uuid\":\"35387513-c312-4a59-ba35-b0c8d1d9e5b2\"},{\"content\":{\"connectorIds\":[\"Out1\"],\"side\":\"RIGHT\"},\"type\":\"ConnectorPlacement.EquallySpacedRectSide\",\"uuid\":\"918617f2-90f0-4ba4-a6a6-e8d81c7788fe\"},{\"content\":{\"connectorIds\":[\"In2\"],\"side\":\"TOP\"},\"type\":\"ConnectorPlacement.EquallySpacedRectSide\",\"uuid\":\"3f5e26f8-529e-48bf-bbb2-eea156dc5bb8\"}]},\"type\":\"ConnectorPlacement.EquallySpacedConnector\",\"uuid\":\"880db2e6-e43a-49ce-ada4-a650fe852eca\"}],\"packageUris\":[\"http://schema.mathworks.com/mf0/Connector/R2020b\"],\"version\":\"1.0\"}"
  Main Controller : Subsystem
      settings: PortSchema="{\"entries\":[{\"content\":{\"sides\":[{\"content\":{\"connectorIds\":[\"In1\",\"In2\",\"In3\"]},\"type\":\"ConnectorPlacement.EquallySpacedRectSide\",\"uuid\":\"8a67eb54-eb6c-45e0-a850-95ec79aece8e\"},{\"content\":{\"connectorIds\":[\"Out1\",\"Out2\",\"Out3\",\"Out4\"],\"side\":\"RIGHT\"},\"type\":\"ConnectorPlacement.EquallySpacedRectSide\",\"uuid\":\"1aa20a3e-bb67-4fbd-b209-2be32aa0ff5f\"},{\"content\":{\"connectorIds\":[\"In4\"],\"side\":\"TOP\"},\"type\":\"ConnectorPlacement.EquallySpacedRectSide\",\"uuid\":\"d9057974-3623-4d09-abc8-3de32842b7f7\"}]},\"type\":\"ConnectorPlacement.EquallySpacedConnector\",\"uuid\":\"e87a5b91-25f0-4827-bb39-498a99db0a00\"}],\"packageUris\":[\"http://schema.mathworks.com/mf0/Connector/R2020b\"],\"version\":\"1.0\"}"
  Reference Supervisor : Subsystem
  FlightControl : Outport
  wires:
  Bus Creator/1 -> FlightControl/1
  Main Controller/1(rollAxis) -> Bus Creator/1  "rollAxis"
  Main Controller/2(pitchAxis) -> Bus Creator/2  "pitchAxis"
  Main Controller/3(yawAxis) -> Bus Creator/3  "yawAxis"
  Main Controller/4(thrustAxis) -> Bus Creator/4  "thrustAxis"
  FlightManagement/1 -> Controller Supervisor/1(FlightManagement), Reference Supervisor/2(FlightManagement)
  EstimatedStates/1 -> Main Controller/2(EstimatedStates), Error Computation/1(EstimatedStates), Reference Supervisor/3(EstimatedStates)
  Error Computation/1(Errors) -> Main Controller/1(Errors)
  Controller Supervisor/1(StateController) -> Main Controller/3(StateController)
  Reference/1 -> Reference Supervisor/1(Reference)
  Reference Supervisor/1(EffectiveReference) -> Main Controller/4(Reference), Error Computation/2(Reference)

== system UAV_Research_Environment/Autopilot/Flight Management ==
  Reference : Inport
  Landed : Inport  Port=2
  OperatorCommands : Inport  Port=3
  EstimatorStatus : Inport  Port=4
  TouchdownCandidate : Inport  Port=5
  Bus Creator : BusCreator  Inputs=4
  Bus Selector : BusSelector  OutputSignals=Complete
  Bus Selector1 : BusSelector  OutputSignals=ArmCommand,RunTrajectoryRequestID
  Bus Selector2 : BusSelector  OutputSignals=NavValid
  Mode Logic : Stateflow chart  TreatAsAtomicUnit=on
      settings: PortSchema="{\"entries\":[{\"content\":{\"sides\":[{\"content\":{\"connectorIds\":[\"In2\",\"In3\",\"In1\",\"In4\",\"In5\",\"In6\"]},\"type\":\"ConnectorPlacement.EquallySpacedRectSide\",\"uuid\":\"788618a1-afde-45fd-a444-c4676f60bd1e\"},{\"content\":{\"connectorIds\":[\"Out1\",\"Out2\",\"Out3\",\"Out4\"],\"side\":\"RIGHT\"},\"type\":\"ConnectorPlacement.EquallySpacedRectSide\",\"uuid\":\"3490d72a-805d-4787-9424-38b278ed593c\"},{\"content\":{\"side\":\"TOP\"},\"type\":\"ConnectorPlacement.EquallySpacedRectSide\",\"uuid\":\"4eec8dce-4ce3-4ba4-8d4f-ef5a5ab16a5a\"}]},\"type\":\"ConnectorPlacement.EquallySpacedConnector\",\"uuid\":\"71fc6e95-058a-40d1-8b99-b127362c140e\"}],\"packageUris\":[\"http://schema.mathworks.com/mf0/Connector/R2020b\"],\"version\":\"1.0\"}"
  FlightManagement : Outport
  wires:
  Reference/1 -> Bus Selector/1
  Bus Selector/1 -> Mode Logic/1(Complete)  "<Complete>"
  Mode Logic/1(mode) -> Bus Creator/1  "mode"
  Mode Logic/2(armed) -> Bus Creator/2  "armed"
  Mode Logic/3(reset) -> Bus Creator/3  "reset"
  Mode Logic/4(missionComplete) -> Bus Creator/4  "missionComplete"
  Bus Creator/1 -> FlightManagement/1
  OperatorCommands/1 -> Bus Selector1/1
  Bus Selector1/2 -> Mode Logic/3(RunTrajectoryRequestID)  "<RunTrajectoryRequestID>"
  Bus Selector1/1 -> Mode Logic/2(ArmCommand)  "<ArmCommand>"
  Landed/1 -> Mode Logic/4(Landed)
  EstimatorStatus/1 -> Bus Selector2/1
  Bus Selector2/1 -> Mode Logic/6(NavValid)  "<NavValid>"
  TouchdownCandidate/1 -> Mode Logic/5(TouchdownCandidate)

== system UAV_Research_Environment/Autopilot/Landed Detector ==
  Reference : Inport
  EstimatorStatus : Inport  Port=2
  OperatorCommands : Inport  Port=3
  EstimatedStates : Inport  Port=4
  Bus Selector : BusSelector  OutputSignals=Position_ref,Complete,Phase
  Bus Selector1 : BusSelector  OutputSignals=Position,Velocity,Attitude.Euler,AngularRate
  Bus Selector2 : BusSelector  OutputSignals=RunTrajectoryRequestID
  Bus Selector3 : BusSelector  OutputSignals=NavValid
  Landing_Confirmation : MATLAB Function  TreatAsAtomicUnit=on
  Landed : Outport
  TouchdownCandidate : Outport  Port=2
  wires:
  Reference/1 -> Bus Selector/1
  EstimatedStates/1 -> Bus Selector1/1
  Landing_Confirmation/1(Landed) -> Landed/1
  Bus Selector1/1 -> Landing_Confirmation/1(Position)  "<Position>"
  Bus Selector1/2 -> Landing_Confirmation/2(Velocity)  "<Velocity>"
  Bus Selector1/4 -> Landing_Confirmation/4(AngularRate)  "<AngularRate>"
  Bus Selector1/3 -> Landing_Confirmation/3(Euler)  "<Euler>"
  Bus Selector/1 -> Landing_Confirmation/5(Position_ref)  "<Position_ref>"
  Bus Selector/2 -> Landing_Confirmation/6(Complete)  "<Complete>"
  OperatorCommands/1 -> Bus Selector2/1
  Bus Selector2/1 -> Landing_Confirmation/8(RunTrajectoryRequestID)  "<RunTrajectoryRequestID>"
  EstimatorStatus/1 -> Bus Selector3/1
  Bus Selector3/1 -> Landing_Confirmation/9(NavValid)  "<NavValid>"
  Landing_Confirmation/2(TouchdownCandidate) -> TouchdownCandidate/1
  [NUM_WAYPOINTS] -> Landing_Confirmation/10(NumWaypoints)
  Bus Selector/3 -> Landing_Confirmation/7(Phase)  "<Phase>"

== system UAV_Research_Environment/Autopilot/Motor Command ==
  MotorCmd : Inport
  FlightManagement : Inport  Port=2
  Armed Idle Omega : Constant  Value=AUTOPILOT.motor.armedIdleOmega_rad_s
  Bus Selector : BusSelector  OutputSignals=mode
  Disarmed Omega : Constant  Value=AUTOPILOT.motor.disarmedOmega_rad_s
  Lower limit : Constant  Value=AUTOPILOT.motor.minOmega_rad_s
  Motor Spool Logic : MATLAB Function  TreatAsAtomicUnit=on
  "Multiport Switch " : MultiPortSwitch  Inputs=7  SaturateOnIntegerOverflow=off  InputSameDT=off
  "Saturation Dynamic " : simulink/Discontinuities/Saturation Dynamic  OutMin=[]  OutMax=[]  OutDataTypeStr=Inherit: Same as second input  OutDataType=fixdt(1, 16)  OutScaling=2^-10  DoSatur=off
  Upper limit : Constant  Value=AUTOPILOT.motor.maxOmega_rad_s
  Omega : Outport
  wires:
  Disarmed Omega/1 -> "Multiport Switch "/2
  Armed Idle Omega/1 -> "Multiport Switch "/3
  MotorCmd/1 -> "Multiport Switch "/5, "Multiport Switch "/6, "Multiport Switch "/8, "Multiport Switch "/7, "Multiport Switch "/4
  FlightManagement/1 -> Bus Selector/1
  Bus Selector/1 -> Motor Spool Logic/1(mode), "Multiport Switch "/1  "<mode>"
  "Multiport Switch "/1 -> Motor Spool Logic/2(u)
  "Saturation Dynamic "/1 -> Omega/1
  Upper limit/1 -> "Saturation Dynamic "/1
  Lower limit/1 -> "Saturation Dynamic "/3
  Motor Spool Logic/1(y) -> "Saturation Dynamic "/2

== system UAV_Research_Environment/Control Ground Station/Mission Manager ==
  RunTrajectoryRequestID : Inport
  Position : Inport  Port=2
  Velocity : Inport  Port=3
  EstimatorStatus : Inport  Port=4
  NumWaypoints : Inport  Port=5
  t : Inport  Port=6
  MissionPlan : Inport  Port=7
  Bus Selector : BusSelector  OutputSignals=NavValid
  Constant : Constant  Value=TRAJECTORY_CONFIG.selectedPassThroughIntermediate
  Mission_Manager : MATLAB Function  TreatAsAtomicUnit=on
  Terminator : Terminator
  TargetPosition : Outport
  TargetYaw : Outport  Port=2
  TargetID : Outport  Port=3
  Phase : Outport  Port=4
  Active : Outport  Port=5
  Complete : Outport  Port=6
  wires:
  t/1 -> Mission_Manager/1(t)
  RunTrajectoryRequestID/1 -> Mission_Manager/2(RunTrajectoryRequestID)
  Position/1 -> Mission_Manager/3(Position)
  Velocity/1 -> Mission_Manager/4(Velocity)
  Mission_Manager/6(Complete) -> Complete/1
  Mission_Manager/5(Active) -> Active/1
  Mission_Manager/4(Phase) -> Phase/1
  Mission_Manager/3(TargetID) -> TargetID/1
  Mission_Manager/2(TargetYaw) -> TargetYaw/1
  Mission_Manager/1(TargetPosition) -> TargetPosition/1
  EstimatorStatus/1 -> Bus Selector/1
  Bus Selector/1 -> Mission_Manager/7(NavValid)  "<NavValid>"
  MissionPlan/1 -> Mission_Manager/5(MissionPlan)
  NumWaypoints/1 -> Mission_Manager/6(NumWaypoints)
  Constant/1 -> Mission_Manager/8(PassThroughIntermediate)
  Mission_Manager/7(MissionDebug) -> Terminator/1

== system UAV_Research_Environment/Control Ground Station/Mission Plan ==
  HomePosition : Inport
  Constant : Constant  Value=TRAJECTORY_CONFIG.selectedMissionPlanBuffer
  Constant1 : Constant  Value=TRAJECTORY_CONFIG.selectedNumWaypoints
  Generate_Mission_Plan : MATLAB Function  TreatAsAtomicUnit=on
  Terminator : Terminator
  MissionPlan : Outport
  NumWaypoints : Outport  Port=2
  wires:
  HomePosition/1 -> Generate_Mission_Plan/1(HomePosition)
  Generate_Mission_Plan/1(MissionPlan) -> MissionPlan/1
  Constant1/1 -> Generate_Mission_Plan/3(NumWaypointsIn)
  Constant/1 -> Generate_Mission_Plan/2(MissionPlanRelative)
  Generate_Mission_Plan/2(NumWaypoints) -> NumWaypoints/1
  Generate_Mission_Plan/3(MissionHome) -> Terminator/1

== system UAV_Research_Environment/Control Ground Station/Waypoint Navigator ==
  t : Inport
  MissionPlan : Inport  Port=2
  TargetPosition : Inport  Port=3
  TargetYaw : Inport  Port=4
  TargetID : Inport  Port=5
  Phase : Inport  Port=6
  Landed : Inport  Port=7
  NumWaypoints : Inport  Port=8
  Waypoint_Navigator : MATLAB Function  TreatAsAtomicUnit=on
  Position_ref : Outport
  Velocity_ref : Outport  Port=2
  Acceleration_ref : Outport  Port=3
  Yaw_ref : Outport  Port=4
  YawRate_ref : Outport  Port=5
  wires:
  t/1 -> Waypoint_Navigator/1(t)
  MissionPlan/1 -> Waypoint_Navigator/2(MissionPlan)
  TargetPosition/1 -> Waypoint_Navigator/3(TargetPosition)
  TargetYaw/1 -> Waypoint_Navigator/4(TargetYaw)
  TargetID/1 -> Waypoint_Navigator/5(TargetID)
  Waypoint_Navigator/1(Position_ref) -> Position_ref/1
  Waypoint_Navigator/2(Velocity_ref) -> Velocity_ref/1
  Waypoint_Navigator/3(Acceleration_ref) -> Acceleration_ref/1
  Waypoint_Navigator/4(Yaw_ref) -> Yaw_ref/1
  Waypoint_Navigator/5(YawRate_ref) -> YawRate_ref/1
  Phase/1 -> Waypoint_Navigator/6(Phase)
  Landed/1 -> Waypoint_Navigator/7(Landed)
  NumWaypoints/1 -> Waypoint_Navigator/8(NumWaypoints)

== system UAV_Research_Environment/Environment/Wind Disturbances ==
  States : Inport
  OFF : Subsystem  VariantControl=DIST_ENABLE == false
  ON : Subsystem  VariantControl=DIST_ENABLE == true
  v_wind : Outport
  w_wind : Outport  Port=2

== system UAV_Research_Environment/Plots & Metrics/Data Logging ==
  EstimatorComparison : Inport
  EstStates : Inport  Port=2
  TrueStates : Inport  Port=3
  Omega : Inport  Port=4
  ControlAxes : Inport  Port=5
  CmdAttitude : Inport  Port=6
  CGS : Inport  Port=7
  CmdAngularRate : Inport  Port=8
  SelectedStates : Inport  Port=9
  "MissionPlan " : Inport  Port=10
  Bus Selector : BusSelector  OutputSignals=Attitude.Euler,AngularRate
  To Workspace : ToWorkspace  VariableName=trueStatesLog  SaveFormat=Timeseries  SampleTime=-1
  To Workspace1 : ToWorkspace  VariableName=estStatesLog  SaveFormat=Timeseries  SampleTime=-1
  To Workspace10 : ToWorkspace  VariableName=MissionPlanLog  SaveFormat=Timeseries  SampleTime=-1
  To Workspace2 : ToWorkspace  VariableName=estimatorComparisonLog  SaveFormat=Timeseries  SampleTime=-1
  To Workspace3 : ToWorkspace  VariableName=cgsLog  SaveFormat=Timeseries  SampleTime=-1
  To Workspace4 : ToWorkspace  VariableName=controlAxesLog  SaveFormat=Timeseries  SampleTime=-1
  To Workspace5 : ToWorkspace  VariableName=cmdAttitudeLog  SaveFormat=Timeseries  SampleTime=-1
  To Workspace6 : ToWorkspace  VariableName=cmdAngularRateLog  SaveFormat=Timeseries  SampleTime=-1
  To Workspace7 : ToWorkspace  VariableName=omegaLog  SaveFormat=Timeseries  SampleTime=-1
  To Workspace8 : ToWorkspace  VariableName=selectedEulerLog  SaveFormat=Timeseries  SampleTime=-1
  To Workspace9 : ToWorkspace  VariableName=selectedAngularRateLog  SaveFormat=Timeseries  SampleTime=-1
  wires:
  TrueStates/1 -> To Workspace/1
  EstimatorComparison/1 -> To Workspace2/1
  EstStates/1 -> To Workspace1/1
  CGS/1 -> To Workspace3/1
  CmdAngularRate/1 -> To Workspace6/1
  CmdAttitude/1 -> To Workspace5/1
  ControlAxes/1 -> To Workspace4/1
  Omega/1 -> To Workspace7/1
  SelectedStates/1 -> Bus Selector/1
  Bus Selector/1 -> To Workspace8/1  "<Euler>"
  Bus Selector/2 -> To Workspace9/1  "<AngularRate>"
  "MissionPlan "/1 -> To Workspace10/1

== system UAV_Research_Environment/Plots & Metrics/Estimator Comparison ==
  True : Inport
  Est : Inport  Port=2
  Bus Creator : BusCreator  Inputs=5
  Bus Creator1 : BusCreator  Inputs=5
  Bus Creator2 : BusCreator  Inputs=2
  Bus Selector : BusSelector  OutputSignals=Position,Velocity,Acceleration,AngularRate,Attitude.Euler,Attitude.Q
  Bus Selector1 : BusSelector  OutputSignals=Position,Velocity,Acceleration,AngularRate,Attitude.Euler,Attitude.Q
  Dot Product{,1..3} (4 alike) : DotProduct  OutDataTypeStr=Inherit: Inherit via internal rule
  Euler_Error : MATLAB Function  TreatAsAtomicUnit=on
  Quaternion_Attitude_Error : MATLAB Function  TreatAsAtomicUnit=on
  Sqrt{,1..3} (4 alike) : Sqrt
  Sum{,1..3} (4 alike) : Sum  Inputs=|-+
  EstimatorComparison : Outport
  wires:
  True/1 -> Bus Selector/1
  Est/1 -> Bus Selector1/1
  Bus Selector/1 -> Sum/1  "<Position>"
  Bus Selector/2 -> Sum1/1  "<Velocity>"
  Bus Selector/3 -> Sum2/1  "<Acceleration>"
  Bus Selector/4 -> Sum3/1  "<AngularRate>"
  Bus Selector1/1 -> Sum/2  "<Position>"
  Bus Selector1/2 -> Sum1/2  "<Velocity>"
  Bus Selector1/3 -> Sum2/2  "<Acceleration>"
  Bus Selector1/4 -> Sum3/2  "<AngularRate>"
  Sum/1 -> Bus Creator1/1, Dot Product/1, Dot Product/2  "PositionError"
  Sum1/1 -> Bus Creator1/2, Dot Product2/1, Dot Product2/2  "VelocityError"
  Sum3/1 -> Bus Creator1/4, Dot Product1/2, Dot Product1/1  "AngularRateError"
  Sum2/1 -> Dot Product3/1, Dot Product3/2, Bus Creator1/3  "AccelerationError"
  Bus Selector/5 -> Euler_Error/1(Euler_true)  "<Euler>"
  Bus Selector1/5 -> Euler_Error/2(Euler_est)  "<Euler>"
  Dot Product/1 -> Sqrt/1
  Sqrt/1 -> Bus Creator/1  "PositionErrorNorm"
  Dot Product1/1 -> Sqrt3/1
  Dot Product2/1 -> Sqrt1/1
  Dot Product3/1 -> Sqrt2/1
  Sqrt1/1 -> Bus Creator/2  "VelocityErrorNorm"
  Sqrt3/1 -> Bus Creator/4  "AngularRateErrorNorm"
  Sqrt2/1 -> Bus Creator/3  "AccelerationErrorNorm"
  Bus Creator/1 -> Bus Creator2/1  "Norms"
  Euler_Error/1(EulerError) -> Bus Creator1/5  "EulerError"
  Bus Creator1/1 -> Bus Creator2/2  "Errors"
  Bus Creator2/1 -> EstimatorComparison/1  "EstimatorComparison"
  Bus Selector/6 -> Quaternion_Attitude_Error/1(Q_true)  "<Q>"
  Bus Selector1/6 -> Quaternion_Attitude_Error/2(Q_est)  "<Q>"
  Quaternion_Attitude_Error/1(AttitudeErrorNorm) -> Bus Creator/5  "AttitudeErrorNorm"
